simulink model "sistemaB"  (R2025b)
settings: Solver=VariableStepAuto  StartTime=0.0  StopTime=10.0  MaxStep=1E-3  RelTol=1e-3
libraries: slpidlib x2
settings DataIOCC: ReturnWorkspaceOutputs=off
settings DebuggingCC: AlgebraicLoopMsg=none  ArtificialAlgebraicLoopMsg=none  MaxConsecutiveZCsMsg=none

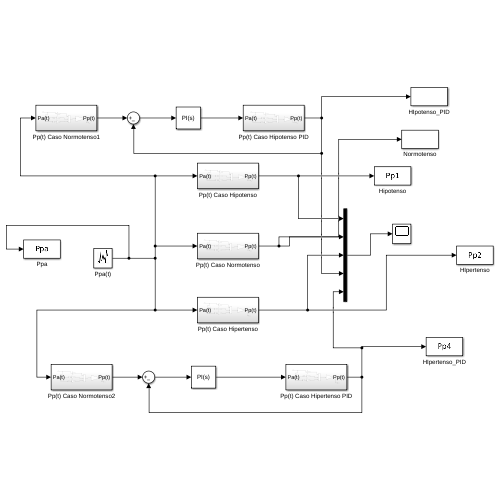
[thumbnail: Simulink's stored preview of the top-level diagram]
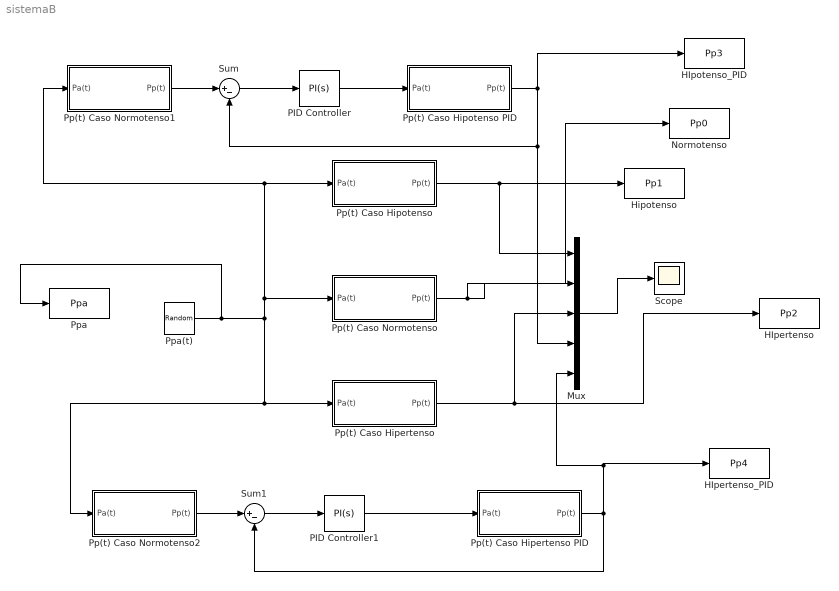
== system sistemaB ==
  HIpertenso : ToWorkspace  VariableName=Pp2  SampleTime=-1
  HIpertenso_PID : ToWorkspace  VariableName=Pp4  SampleTime=-1
  HIpotenso_PID : ToWorkspace  VariableName=Pp3  SampleTime=-1
  Hipotenso : ToWorkspace  VariableName=Pp1  SampleTime=-1
  Mux : Mux  Inputs=5
  Normotenso : ToWorkspace  VariableName=Pp0  SampleTime=-1
  PID Controller : slpidlib/PID Controller  Controller=PI  Form=Parallel  TimeDomain=Continuous-time  UseExternalTs=off  SampleTime=-1  IntegratorMethod=Forward Euler  FilterMethod=Forward Euler  ControllerParametersSource=internal  P=0.0001033333  I=41686938.2080771  UseKiTs=off  D=0  UseExternalDerivativeSource=off  N=100  UseFilter=on  TunerSelectOption=Transfer Function Based (PID Tuner App)  InitialConditionSource=internal  InitialConditionForIntegrator=0  InitialConditionForFilter=0  DifferentiatorICPrevScaledInput=0  ExternalReset=none  TrackingMode=off  Kt=1  LimitOutput=off  SatLimitsSource=internal  UpperSaturationLimit=inf  LowerSaturationLimit=-inf  LinearizeAsGain=on  AntiWindupMode=none  Kb=1  LimitIntegrator=off  UpperIntegratorSaturationLimit=inf  LowerIntegratorSaturationLimit=-inf  POutMin=[]  POutMax=[]  IOutMin=[]  IOutMax=[]  DOutMin=[]  DOutMax=[]  NOutMin=[]  NOutMax=[]  SumOutMin=[]  SumOutMax=[]  SaturationOutMin=[]  SaturationOutMax=[]  PParamMin=[]  PParamMax=[]  IParamMin=[]  IParamMax=[]  DParamMin=[]  DParamMax=[]  NParamMin=[]  NParamMax=[]  KbParamMin=[]  KbParamMax=[]  KtParamMin=[]  KtParamMax=[]  KbOutMin=[]  KbOutMax=[]  KtOutMin=[]  KtOutMax=[]  IntegratorOutMin=[]  IntegratorOutMax=[]  FilterOutMin=[]  FilterOutMax=[]  SumI1OutMin=[]  SumI1OutMax=[]  SumI2OutMin=[]  SumI2OutMax=[]  SumI3OutMin=[]  SumI3OutMax=[]  SumI4OutMin=[]  SumI4OutMax=[]  SumDOutMin=[]  SumDOutMax=[]  DifferentiatorOutMin=[]  DifferentiatorOutMax=[]  FilterDiffOutCoefMin=[]  FilterDiffOutCoefMax=[]  ReciprocalOutMin=[]  ReciprocalOutMax=[]  SumDenOutMin=[]  SumDenOutMax=[]  SumNumOutMin=[]  SumNumOutMax=[]  DivideOutMin=[]  DivideOutMax=[]  UdiffTsProdOutMin=[]  UdiffTsProdOutMax=[]  NTsProdOutMin=[]  NTsProdOutMax=[]  UintegralTsProdOutMin=[]  UintegralTsProdOutMax=[]  UngainTsProdOutMin=[]  UngainTsProdOutMax=[]  ClampingZeroOutDataTypeStr=Inherit: Inherit via back propagation  ClampingZeroOutMin=[]  ClampingZeroOutMax=[]  FilterDenConstantOutDataTypeStr=Inherit: Inherit via back propagation  FilterDenConstantOutMin=[]  FilterDenConstantOutMax=[]  PCopyOutDataTypeStr=Inherit: Inherit via back propagation  PCopyOutMin=[]  PCopyOutMax=[]  NCopyOutDataTypeStr=Inherit: Inherit via back propagation  NCopyOutMin=[]  NCopyOutMax=[]  IntegratorContinuousStateAttributes=''  IntegratorStateMustResolveToSignalObject=off  IntegratorRTWStateStorageClass=Auto  FilterContinuousStateAttributes=''  FilterStateMustResolveToSignalObject=off  FilterRTWStateStorageClass=Auto  ParallelPVariant=InternalParameters  IdealPVariant=Disabled  IVariant=InternalParameters  DVariant=Disabled  IntegratorVariant=Continuous  SatVariant=Disabled  AWVariant=Passthrough  PCopyVariant=Disabled  TRVariant=Disabled  FdbkBlocksVariant=Forward  IdealPFdbkVariant=Disabled  SatFdbkVariant=Disabled  DerivativeFilterVariant=Disabled  NVariant=Disabled  NCopyVariant=Disabled_SignalSpec  FilterICVariant=Disabled  IntegratorICVariant=InternalICs  ExternalResetVariant=Disabled  TRSumVariant=Passthrough  SumFdbkVariant=Disabled  SumVariant=Sum_PI  TsampFilterVariant=InternalTs  TsampNgainVariant=Passthrough  TsampIntegralVariant=Disabled_SignalSpec  ExternalSaturationOutDataTypeStr=Inherit: Same as second input  DerivativeSourceVariant=Disabled  PreIntVariant=InternalPreInt
  PID Controller1 : slpidlib/PID Controller  Controller=PI  Form=Parallel  TimeDomain=Continuous-time  UseExternalTs=off  SampleTime=-1  IntegratorMethod=Forward Euler  FilterMethod=Forward Euler  ControllerParametersSource=internal  P=10  I=4132.36404565657  UseKiTs=off  D=0  UseExternalDerivativeSource=off  N=100  UseFilter=on  TunerSelectOption=Transfer Function Based (PID Tuner App)  InitialConditionSource=internal  InitialConditionForIntegrator=0  InitialConditionForFilter=0  DifferentiatorICPrevScaledInput=0  ExternalReset=none  TrackingMode=off  Kt=1  LimitOutput=off  SatLimitsSource=internal  UpperSaturationLimit=inf  LowerSaturationLimit=-inf  LinearizeAsGain=on  AntiWindupMode=none  Kb=1  LimitIntegrator=off  UpperIntegratorSaturationLimit=inf  LowerIntegratorSaturationLimit=-inf  POutMin=[]  POutMax=[]  IOutMin=[]  IOutMax=[]  DOutMin=[]  DOutMax=[]  NOutMin=[]  NOutMax=[]  SumOutMin=[]  SumOutMax=[]  SaturationOutMin=[]  SaturationOutMax=[]  PParamMin=[]  PParamMax=[]  IParamMin=[]  IParamMax=[]  DParamMin=[]  DParamMax=[]  NParamMin=[]  NParamMax=[]  KbParamMin=[]  KbParamMax=[]  KtParamMin=[]  KtParamMax=[]  KbOutMin=[]  KbOutMax=[]  KtOutMin=[]  KtOutMax=[]  IntegratorOutMin=[]  IntegratorOutMax=[]  FilterOutMin=[]  FilterOutMax=[]  SumI1OutMin=[]  SumI1OutMax=[]  SumI2OutMin=[]  SumI2OutMax=[]  SumI3OutMin=[]  SumI3OutMax=[]  SumI4OutMin=[]  SumI4OutMax=[]  SumDOutMin=[]  SumDOutMax=[]  DifferentiatorOutMin=[]  DifferentiatorOutMax=[]  FilterDiffOutCoefMin=[]  FilterDiffOutCoefMax=[]  ReciprocalOutMin=[]  ReciprocalOutMax=[]  SumDenOutMin=[]  SumDenOutMax=[]  SumNumOutMin=[]  SumNumOutMax=[]  DivideOutMin=[]  DivideOutMax=[]  UdiffTsProdOutMin=[]  UdiffTsProdOutMax=[]  NTsProdOutMin=[]  NTsProdOutMax=[]  UintegralTsProdOutMin=[]  UintegralTsProdOutMax=[]  UngainTsProdOutMin=[]  UngainTsProdOutMax=[]  ClampingZeroOutDataTypeStr=Inherit: Inherit via back propagation  ClampingZeroOutMin=[]  ClampingZeroOutMax=[]  FilterDenConstantOutDataTypeStr=Inherit: Inherit via back propagation  FilterDenConstantOutMin=[]  FilterDenConstantOutMax=[]  PCopyOutDataTypeStr=Inherit: Inherit via back propagation  PCopyOutMin=[]  PCopyOutMax=[]  NCopyOutDataTypeStr=Inherit: Inherit via back propagation  NCopyOutMin=[]  NCopyOutMax=[]  IntegratorContinuousStateAttributes=''  IntegratorStateMustResolveToSignalObject=off  IntegratorRTWStateStorageClass=Auto  FilterContinuousStateAttributes=''  FilterStateMustResolveToSignalObject=off  FilterRTWStateStorageClass=Auto  ParallelPVariant=InternalParameters  IdealPVariant=Disabled  IVariant=InternalParameters  DVariant=Disabled  IntegratorVariant=Continuous  SatVariant=Disabled  AWVariant=Passthrough  PCopyVariant=Disabled  TRVariant=Disabled  FdbkBlocksVariant=Forward  IdealPFdbkVariant=Disabled  SatFdbkVariant=Disabled  DerivativeFilterVariant=Disabled  NVariant=Disabled  NCopyVariant=Disabled_SignalSpec  FilterICVariant=Disabled  IntegratorICVariant=InternalICs  ExternalResetVariant=Disabled  TRSumVariant=Passthrough  SumFdbkVariant=Disabled  SumVariant=Sum_PI  TsampFilterVariant=InternalTs  TsampNgainVariant=Passthrough  TsampIntegralVariant=Disabled_SignalSpec  ExternalSaturationOutDataTypeStr=Inherit: Same as second input  DerivativeSourceVariant=Disabled  PreIntVariant=InternalPreInt
  Pp(t) Caso Hipertenso : Subsystem
  Pp(t) Caso Hipertenso PID : Subsystem
  Pp(t) Caso Hipotenso : Subsystem
  Pp(t) Caso Hipotenso PID : Subsystem
  Pp(t) Caso Normotenso : Subsystem
  Pp(t) Caso Normotenso1 : Subsystem
  Pp(t) Caso Normotenso2 : Subsystem
  Ppa : ToWorkspace  VariableName=Ppa  SampleTime=-1
  Ppa(t) : UniformRandomNumber  Minimum=-0.2  Seed=106  SampleTime=0.5
  Scope : Scope
      settings: ActiveDisplayYMinimum=-0.27959675969936537  ActiveDisplayYMaximum=1.2309691111384318
  Sum : Sum  Inputs=|+-
  Sum1 : Sum  Inputs=|+-
  wires:
  Pp(t) Caso Hipotenso/1(Pp(t)) -> Hipotenso/1, Mux/1
  Mux/1 -> Scope/1
  Pp(t) Caso Normotenso/1(Pp(t)) -> Normotenso/1, Mux/2
  Pp(t) Caso Hipertenso/1(Pp(t)) -> HIpertenso/1, Mux/3
  Ppa(t)/1 -> Ppa/1, Pp(t) Caso Normotenso2/1(Pa(t)), Pp(t) Caso Hipertenso/1(Pa(t)), Pp(t) Caso Normotenso/1(Pa(t)), Pp(t) Caso Normotenso1/1(Pa(t)), Pp(t) Caso Hipotenso/1(Pa(t))
  Pp(t) Caso Normotenso1/1(Pp(t)) -> Sum/1
  Sum/1 -> PID Controller/1
  PID Controller/1 -> Pp(t) Caso Hipotenso PID/1(Pa(t))
  Pp(t) Caso Hipotenso PID/1(Pp(t)) -> Mux/4, Sum/2, HIpotenso_PID/1
  Pp(t) Caso Normotenso2/1(Pp(t)) -> Sum1/1
  Sum1/1 -> PID Controller1/1
  PID Controller1/1 -> Pp(t) Caso Hipertenso PID/1(Pa(t))
  Pp(t) Caso Hipertenso PID/1(Pp(t)) -> HIpertenso_PID/1, Mux/5, Sum1/2

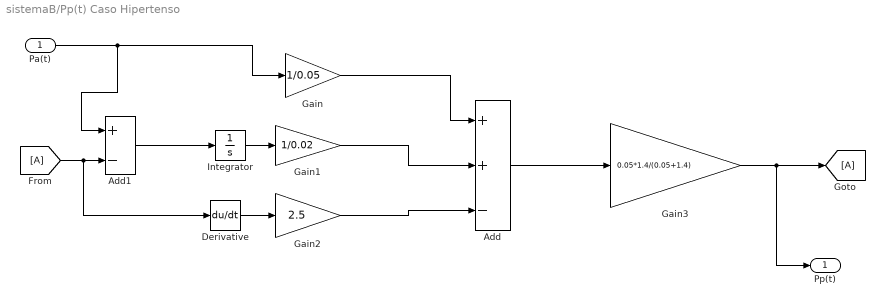
== system sistemaB/Pp(t) Caso Hipertenso ==
  Pa(t) : Inport
  Add : Sum  Inputs=++-
  Add1 : Sum  Inputs=+-
  Derivative : Derivative
  From : From
  Gain : Gain  Gain=1/0.05
  Gain1 : Gain  Gain=1/0.02
  Gain2 : Gain  Gain=2.5
  Gain3 : Gain  Gain=0.05*1.4/(0.05+1.4)
  Goto : Goto
  Integrator : Integrator
  Pp(t) : Outport
  wires:
  Add/1 -> Gain3/1
  Gain/1 -> Add/1
  Pa(t)/1 -> Add1/1, Gain/1
  Integrator/1 -> Gain1/1
  Add1/1 -> Integrator/1
  Gain3/1 -> Pp(t)/1, Goto/1
  Gain2/1 -> Add/3
  Gain1/1 -> Add/2
  Derivative/1 -> Gain2/1
  From/1 -> Derivative/1, Add1/2

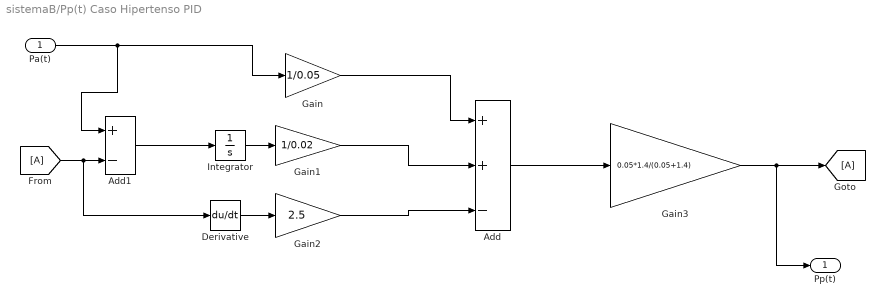
== system sistemaB/Pp(t) Caso Hipertenso PID ==
  Pa(t) : Inport
  Add : Sum  Inputs=++-
  Add1 : Sum  Inputs=+-
  Derivative : Derivative
  From : From
  Gain : Gain  Gain=1/0.05
  Gain1 : Gain  Gain=1/0.02
  Gain2 : Gain  Gain=2.5
  Gain3 : Gain  Gain=0.05*1.4/(0.05+1.4)
  Goto : Goto
  Integrator : Integrator
  Pp(t) : Outport
  wires:
  Add/1 -> Gain3/1
  Gain/1 -> Add/1
  Pa(t)/1 -> Add1/1, Gain/1
  Integrator/1 -> Gain1/1
  Add1/1 -> Integrator/1
  Gain3/1 -> Pp(t)/1, Goto/1
  Gain2/1 -> Add/3
  Gain1/1 -> Add/2
  Derivative/1 -> Gain2/1
  From/1 -> Derivative/1, Add1/2

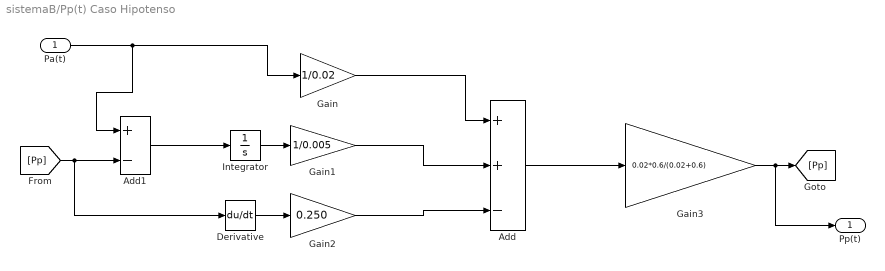
== system sistemaB/Pp(t) Caso Hipotenso ==
  Pa(t) : Inport
  Add : Sum  Inputs=++-
  Add1 : Sum  Inputs=+-
  Derivative : Derivative
  Gain : Gain  Gain=1/0.02
  Gain1 : Gain  Gain=1/0.005
  Gain2 : Gain  Gain=0.250
  Gain3 : Gain  Gain=0.02*0.6/(0.02+0.6)
  Integrator : Integrator
  Pp(t) : Outport
  wires:
  Gain/1 -> Add/1
  Gain1/1 -> Add/2
  Gain2/1 -> Add/3
  Add/1 -> Gain3/1
  Derivative/1 -> Gain2/1
  Integrator/1 -> Gain1/1
  Add1/1 -> Integrator/1
  Pa(t)/1 -> Add1/1, Gain/1
  [Pp] -> Derivative/1, Add1/2
  Gain3/1 -> Pp(t)/1, [Pp]

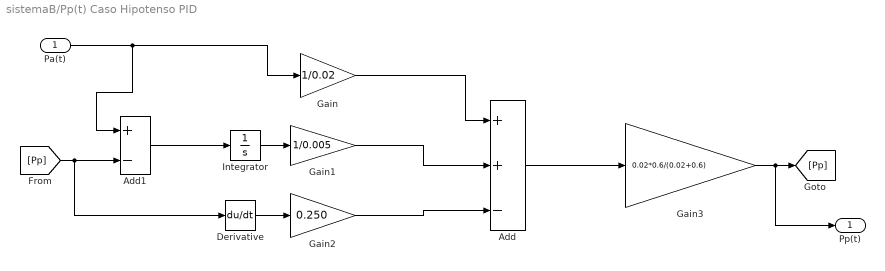
== system sistemaB/Pp(t) Caso Hipotenso PID ==
  Pa(t) : Inport
  Add : Sum  Inputs=++-
  Add1 : Sum  Inputs=+-
  Derivative : Derivative
  Gain : Gain  Gain=1/0.02
  Gain1 : Gain  Gain=1/0.005
  Gain2 : Gain  Gain=0.250
  Gain3 : Gain  Gain=0.02*0.6/(0.02+0.6)
  Integrator : Integrator
  Pp(t) : Outport
  wires:
  Gain/1 -> Add/1
  Gain1/1 -> Add/2
  Gain2/1 -> Add/3
  Add/1 -> Gain3/1
  Derivative/1 -> Gain2/1
  Integrator/1 -> Gain1/1
  Add1/1 -> Integrator/1
  Pa(t)/1 -> Add1/1, Gain/1
  [Pp] -> Derivative/1, Add1/2
  Gain3/1 -> Pp(t)/1, [Pp]

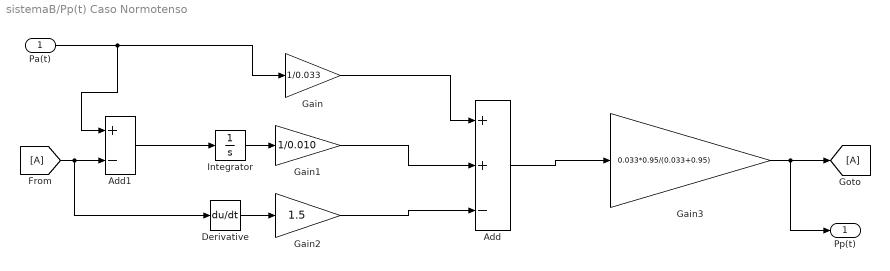
== system sistemaB/Pp(t) Caso Normotenso ==
  Pa(t) : Inport
  Add : Sum  Inputs=++-
  Add1 : Sum  Inputs=+-
  Derivative : Derivative
  From : From
  Gain : Gain  Gain=1/0.033
  Gain1 : Gain  Gain=1/0.010
  Gain2 : Gain  Gain=1.5
  Gain3 : Gain  Gain=0.033*0.95/(0.033+0.95)
  Goto : Goto
  Integrator : Integrator
  Pp(t) : Outport
  wires:
  Add/1 -> Gain3/1
  Gain/1 -> Add/1
  Pa(t)/1 -> Add1/1, Gain/1
  Integrator/1 -> Gain1/1
  Add1/1 -> Integrator/1
  Gain3/1 -> Pp(t)/1, Goto/1
  Gain2/1 -> Add/3
  Gain1/1 -> Add/2
  Derivative/1 -> Gain2/1
  From/1 -> Derivative/1, Add1/2

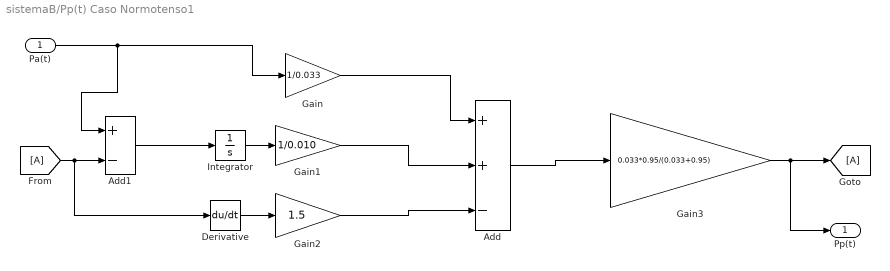
== system sistemaB/Pp(t) Caso Normotenso1 ==
  Pa(t) : Inport
  Add : Sum  Inputs=++-
  Add1 : Sum  Inputs=+-
  Derivative : Derivative
  From : From
  Gain : Gain  Gain=1/0.033
  Gain1 : Gain  Gain=1/0.010
  Gain2 : Gain  Gain=1.5
  Gain3 : Gain  Gain=0.033*0.95/(0.033+0.95)
  Goto : Goto
  Integrator : Integrator
  Pp(t) : Outport
  wires:
  Add/1 -> Gain3/1
  Gain/1 -> Add/1
  Pa(t)/1 -> Add1/1, Gain/1
  Integrator/1 -> Gain1/1
  Add1/1 -> Integrator/1
  Gain3/1 -> Pp(t)/1, Goto/1
  Gain2/1 -> Add/3
  Gain1/1 -> Add/2
  Derivative/1 -> Gain2/1
  From/1 -> Derivative/1, Add1/2

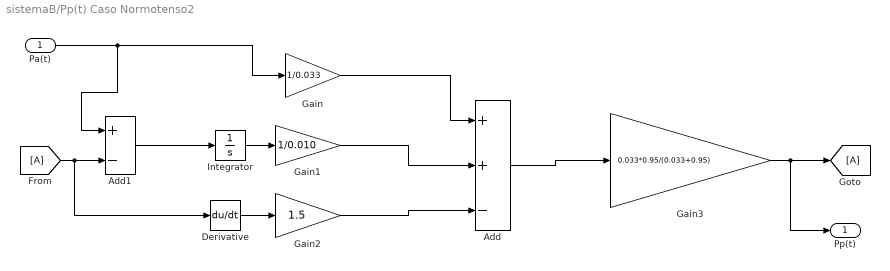
== system sistemaB/Pp(t) Caso Normotenso2 ==
  Pa(t) : Inport
  Add : Sum  Inputs=++-
  Add1 : Sum  Inputs=+-
  Derivative : Derivative
  From : From
  Gain : Gain  Gain=1/0.033
  Gain1 : Gain  Gain=1/0.010
  Gain2 : Gain  Gain=1.5
  Gain3 : Gain  Gain=0.033*0.95/(0.033+0.95)
  Goto : Goto
  Integrator : Integrator
  Pp(t) : Outport
  wires:
  Add/1 -> Gain3/1
  Gain/1 -> Add/1
  Pa(t)/1 -> Add1/1, Gain/1
  Integrator/1 -> Gain1/1
  Add1/1 -> Integrator/1
  Gain3/1 -> Pp(t)/1, Goto/1
  Gain2/1 -> Add/3
  Gain1/1 -> Add/2
  Derivative/1 -> Gain2/1
  From/1 -> Derivative/1, Add1/2
